simulink model "GFLIB_ControllerPIDpAW_BAM"  (Simulink 8.3)
settings: Solver=ode45  StartTime=0.0  StopTime=10.0  RelTol=1e-3
undefined symbols (not defined in the file): f32DerivGain, f32FiltCoef, f32IntegGain, f32PropGain, s16DerivGainShift, s16IntegGainShift, s16PropGainShift
settings Model: Creator=nxf41029  LastModifiedBy=nxf41029
settings DataIOCC: SignalLoggingSaveFormat=Dataset
settings DebuggingCC: UnderspecifiedInitializationDetection=Simplified  StateNameClashWarn=none
settings GRTTargetCC: CombineOutputUpdateFcns=on  GRTInterface=off

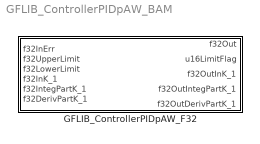
== system GFLIB_ControllerPIDpAW_BAM ==
  GFLIB_ControllerPIDpAW_F32 : Subsystem  mask(GFLIB_ControllerPIDpAW_F32){f32PropGain=f32PropGain, s16PropGainShift=s16PropGainShift, f32IntegGain=f32IntegGain, s16IntegGainShift=s16IntegGainShift, f32DerivGain=f32DerivGain, s16DerivGainShift=s16DerivGainShift, f32FiltCoef=f32FiltCoef}
      mask help: Bit accurate model of parallel form PID controller. All parameters as well as input and output are 32-bit integers except for s16xxxGainShift parameters which are 16-bit signed integers.
      mask init:
      | pos = get_param(gcb, 'Position');width = pos(3) - pos(1); height = pos(4) - pos(2);tX=width/2;tY=height*0.9;
      mask Display: color('black');port_label('input',1,'f32InErr');port_label('input',2,'f32UpperLimit');port_label('input',3,'f32LowerLimit');port_label('input',4,'f32InK_1');port_label('input',5,'f32IntegPartK_1');port_label('input',6,'f32DerivPartK_1');port_label('output',1,'f32Out');port_label('output',2,'u16LimitFlag');port_label('output',3,'f32OutInK_1');port_label('output',4,'f32OutIntegPartK_1');port_label('output',5,'f32OutDerivPartK_1');color('black');disp('GFLIB_ControllerPIDpAW_F32');color('blue');text(tX,tY, 'BAM', 'horizontalAlignment', 'center');

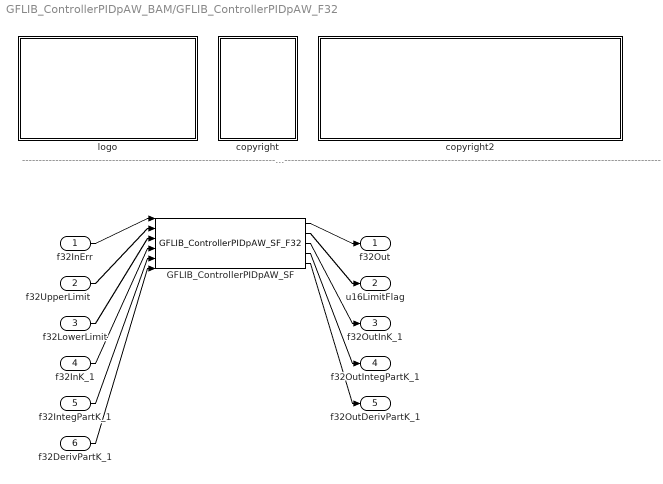
== system GFLIB_ControllerPIDpAW_BAM/GFLIB_ControllerPIDpAW_F32 ==
  note: ---------------------------------------------------------------------------------------------------------------------------------------------------------------------------------------------------
  f32InErr : Inport
  f32UpperLimit : Inport  Port=2
  f32LowerLimit : Inport  Port=3
  f32InK_1 : Inport  Port=4
  f32IntegPartK_1 : Inport  Port=5
  f32DerivPartK_1 : Inport  Port=6
  GFLIB_ControllerPIDpAW_SF : S-Function  FunctionName=GFLIB_ControllerPIDpAW_SF_F32  Parameters=f32PropGain,s16PropGainShift,f32IntegGain,s16IntegGainShift,f32DerivGain,s16DerivGainShift,f32FiltCoef  EnableBusSupport=off
  copyright : Subsystem
      mask Display: text(10,90,'FILE:');text(10,75,'DESRIPTION:');text(10,60,'COPYRIGHT:');text(10,45,'VERSION:');text(10,30,'DATE:')
  copyright2 : Subsystem
      mask Display: text(10,90,'GFLIB_ControllerPIDpAW_BAM_F32.mdl');text(10,75,'Parallel form of a standard PID controller with implemented anti-windup.');text(10,60,'NXP');text(10,45,'0.1');text(10,30,'21-Nov-2018');
  logo : Subsystem
      mask Display: image(imread('logo.jpg'))
  f32Out : Outport
  u16LimitFlag : Outport  Port=2
  f32OutInK_1 : Outport  Port=3
  f32OutIntegPartK_1 : Outport  Port=4
  f32OutDerivPartK_1 : Outport  Port=5
  wires:
  f32InErr/1 -> GFLIB_ControllerPIDpAW_SF/1
  f32UpperLimit/1 -> GFLIB_ControllerPIDpAW_SF/2
  f32LowerLimit/1 -> GFLIB_ControllerPIDpAW_SF/3
  f32InK_1/1 -> GFLIB_ControllerPIDpAW_SF/4
  f32IntegPartK_1/1 -> GFLIB_ControllerPIDpAW_SF/5
  f32DerivPartK_1/1 -> GFLIB_ControllerPIDpAW_SF/6
  GFLIB_ControllerPIDpAW_SF/1 -> f32Out/1
  GFLIB_ControllerPIDpAW_SF/2 -> u16LimitFlag/1
  GFLIB_ControllerPIDpAW_SF/3 -> f32OutInK_1/1
  GFLIB_ControllerPIDpAW_SF/4 -> f32OutIntegPartK_1/1
  GFLIB_ControllerPIDpAW_SF/5 -> f32OutDerivPartK_1/1

== system GFLIB_ControllerPIDpAW_BAM/GFLIB_ControllerPIDpAW_F32/copyright ==

== system GFLIB_ControllerPIDpAW_BAM/GFLIB_ControllerPIDpAW_F32/copyright2 ==

== system GFLIB_ControllerPIDpAW_BAM/GFLIB_ControllerPIDpAW_F32/logo ==
